simulink model "CHEM_FULL_BENCHMARK"  (R2019a)
settings: Solver=FixedStepAuto  StartTime=0.0  StopTime=app.SimuTime  FixedStep=Te  RelTol=1e-3  EnableMultiTasking=on
values from neighbouring files (symbols this model uses):
  A1 = 0.0154    [INIT_FULL.m]    (also in run.m)
  A2 = 0.0154    [INIT_FULL.m]    (also in run.m)
  app = interface    [INIT_FULL.m]    (also in run.m)
  Cvb = 1.5938*1e-4    (= 0.00015938)    [INIT_FULL.m]    (also in run.m)
  Cvo = 1.59640*1e-4    (= 0.00015964)    [INIT_FULL.m]    (also in run.m)
  g = 9.81    [INIT_FULL.m]    (also in run.m)
  h1c = 0.5    [INIT_FULL.m]    (also in run.m)
  h1c_0 = 0    [INIT_FULL.m]    (also in run.m)
  h1max = 0.6    [INIT_FULL.m]    (also in run.m)
  h2c_0 = 0    [INIT_FULL.m]    (also in Variables_Update.m = app.InitialwaterlevelinT206EditField.Value; run.m)
  h2c_max = 0.11    [INIT_FULL.m]    (also in run.m)
  h2c_min = 0.09    [INIT_FULL.m]    (also in run.m)
  h2max = 0.6    [INIT_FULL.m]    (also in run.m)
  Ki = 5*1e-6    (= 5e-06)    [INIT_FULL.m]    (also in run.m)
  Kp = 1e-3    (= 0.001)    [INIT_FULL.m]    (also in run.m)
  Patm = 101325    [INIT_FULL.m]    (also in run.m)
  Qf1 = 1e-4    (= 0.0001)    [INIT_FULL.m]    (also in Variables_Update.m = app.FlowleakfromT1m3sEditField.Value; run.m)
  Qf2 = 1e-4    (= 0.0001)    [INIT_FULL.m]    (also in Variables_Update.m = app.FlowleakfromT2m3sEditField.Value; run.m)
  Qof1 = 1e-4    (= 0.0001)    [INIT_FULL.m]    (also in Variables_Update.m = app.OverflowrateinT1m3sEditField.Value; run.m)
  Qpmax = 1e-2    (= 0.01)    [INIT_FULL.m]    (also in run.m)
  rate_noise_mQp = 0.01*1e-5    (= 1e-07)    [INIT_FULL.m]    (also in run.m)
  rate_noise_mUp = 0.01*1e-5    (= 1e-07)    [INIT_FULL.m]    (also in run.m)
  rate_noise_my1 = 0.5*0.001    (= 0.0005)    [INIT_FULL.m]    (also in run.m)
  rate_noise_my2 = 0.3*0.001    (= 0.0003)    [INIT_FULL.m]    (also in run.m)
  ro = 1000    [INIT_FULL.m]    (also in run.m)
  seed = randi(10000000)    [INIT_FULL.m]    (also in run.m)
  Te = 1    [INIT_FULL.m]    (also in run.m)
  yo = 0    [INIT_FULL.m]    (also in run.m)
(part 2 of 12)

== system CHEM_FULL_BENCHMARK/T2 hidden long theft/Process ==
  note: y2
  note: y1
  note: Ub
  note: Up
  note: Qvo
      | To users
  note: Qp
  note: Qvb
  Constant : Constant  Value=yo
  Subsystem1 : Subsystem
      mask Display: disp('TANK 1')
  Subsystem10 : Subsystem
      mask Display: disp('Sensor\n y2')
  Subsystem11 : Subsystem
      mask Display: disp('Controller 1')
  Subsystem12 : Subsystem
      mask Display: disp('Sensor\n Ub')
  Subsystem13 : Subsystem
      mask Display: disp('Sensor\n Up')
  Subsystem14 : Subsystem
      mask Display: disp('Sensor\n Qp')
  Subsystem15 : Subsystem
      mask Display: disp('Sensor\n P2')
  Subsystem2 : Subsystem
      mask Display: disp('Valve B')
  Subsystem3 : Subsystem
      mask Display: disp('Valve O')
  Subsystem4 : Subsystem
      mask Display: disp('Controller2')
  Subsystem5 : Subsystem
      mask Display: disp('Sensor\n P1')
  Subsystem6 : Subsystem
      mask Display: disp('Pump')
  Subsystem7 : Subsystem
      mask Display: disp('Sensor\n y1')
  Subsystem8 : Subsystem
      mask Display: disp('TANK 2')
  Subsystem9 : Subsystem
      mask Display: disp('OPERATOR\nSET')
  mQp : Outport
  mUb : Outport  Port=2
  "Uo " : Outport  Port=3
  my1 : Outport  Port=4
  my2 : Outport  Port=5
  h1c : Outport  Port=6
  mUp : Outport  Port=7
  mq0 : Outport  Port=8
  y1 : Outport  Port=9
  vol1 : Outport  Port=10
  y2 : Outport  Port=11
  vol2 : Outport  Port=12
  mP1 : Outport  Port=13
  mP2 : Outport  Port=14
  wires:
  Subsystem12/1(mUb) -> mUb/1
  Subsystem3/1(Qv0) -> mq0/1, Subsystem8/1(Qvo)
  Constant/1 -> Subsystem3/3(y0)
  Subsystem13/1(mUp) -> mUp/1
  Subsystem2/1(QVb) -> Subsystem8/2(Qvb), Subsystem1/2(Qvb)
  Subsystem11/1(mUp) -> Subsystem13/1(Up), Subsystem6/1(Up)
  Subsystem9/1(Out3) -> Subsystem11/1(h1c), h1c/1
  Subsystem9/2(Out1) -> "Uo "/1, Subsystem3/1(U0)
  Subsystem7/1(Out5) -> Subsystem11/2(my1), my1/1
  Subsystem14/1(mQp) -> mQp/1
  Subsystem4/1(Out5) -> Subsystem12/1(Ub), Subsystem2/1(Ub)
  Subsystem10/1(my2) -> my2/1, Subsystem4/1(In2)
  Subsystem6/1(mUp) -> Subsystem1/1(Qp), Subsystem14/1(Qp)
  Subsystem7/2(Out1) -> y1/1
  Subsystem7/3(Out2) -> vol1/1
  Subsystem10/2(yy2) -> y2/1
  Subsystem10/3(vol2) -> vol2/1
  Subsystem5/1(mP1) -> mP1/1
  Subsystem1/1(y1) -> Subsystem5/1(y1), Subsystem2/2(y1), Subsystem7/1(In1)
  Subsystem15/1(mP2) -> mP2/1
  Subsystem8/1(y2) -> Subsystem3/2(y2), Subsystem15/1(y2), Subsystem2/3(y2), Subsystem10/1(y2)

== system CHEM_FULL_BENCHMARK/T2 hidden short theft/Process ==
  note: y2
  note: y1
  note: Ub
  note: Up
  note: Qvo
      | To users
  note: Qp
  note: Qvb
  Constant : Constant  Value=yo
  Subsystem1 : Subsystem
      mask Display: disp('TANK 1')
  Subsystem10 : Subsystem
      mask Display: disp('Sensor\n y2')
  Subsystem11 : Subsystem
      mask Display: disp('Controller 1')
  Subsystem12 : Subsystem
      mask Display: disp('Sensor\n Ub')
  Subsystem13 : Subsystem
      mask Display: disp('Sensor\n Up')
  Subsystem14 : Subsystem
      mask Display: disp('Sensor\n Qp')
  Subsystem15 : Subsystem
      mask Display: disp('Sensor\n P2')
  Subsystem2 : Subsystem
      mask Display: disp('Valve B')
  Subsystem3 : Subsystem
      mask Display: disp('Valve O')
  Subsystem4 : Subsystem
      mask Display: disp('Controller2')
  Subsystem5 : Subsystem
      mask Display: disp('Sensor\n P1')
  Subsystem6 : Subsystem
      mask Display: disp('Pump')
  Subsystem7 : Subsystem
      mask Display: disp('Sensor\n y1')
  Subsystem8 : Subsystem
      mask Display: disp('TANK 2')
  Subsystem9 : Subsystem
      mask Display: disp('OPERATOR\nSET')
  mQp : Outport
  mUb : Outport  Port=2
  "Uo " : Outport  Port=3
  my1 : Outport  Port=4
  my2 : Outport  Port=5
  h1c : Outport  Port=6
  mUp : Outport  Port=7
  mq0 : Outport  Port=8
  y1 : Outport  Port=9
  vol1 : Outport  Port=10
  y2 : Outport  Port=11
  vol2 : Outport  Port=12
  mP1 : Outport  Port=13
  mP2 : Outport  Port=14
  wires:
  Subsystem12/1(mUb) -> mUb/1
  Subsystem3/1(Qv0) -> mq0/1, Subsystem8/1(Qvo)
  Constant/1 -> Subsystem3/3(y0)
  Subsystem13/1(mUp) -> mUp/1
  Subsystem2/1(QVb) -> Subsystem8/2(Qvb), Subsystem1/2(Qvb)
  Subsystem11/1(mUp) -> Subsystem13/1(Up), Subsystem6/1(Up)
  Subsystem9/1(Out3) -> Subsystem11/1(h1c), h1c/1
  Subsystem9/2(Out1) -> "Uo "/1, Subsystem3/1(U0)
  Subsystem7/1(Out5) -> Subsystem11/2(my1), my1/1
  Subsystem14/1(mQp) -> mQp/1
  Subsystem4/1(Out5) -> Subsystem12/1(Ub), Subsystem2/1(Ub)
  Subsystem10/1(my2) -> my2/1, Subsystem4/1(In2)
  Subsystem6/1(mUp) -> Subsystem1/1(Qp), Subsystem14/1(Qp)
  Subsystem7/2(Out1) -> y1/1
  Subsystem7/3(Out2) -> vol1/1
  Subsystem10/2(yy2) -> y2/1
  Subsystem10/3(vol2) -> vol2/1
  Subsystem5/1(mP1) -> mP1/1
  Subsystem1/1(y1) -> Subsystem5/1(y1), Subsystem2/2(y1), Subsystem7/1(In1)
  Subsystem15/1(mP2) -> mP2/1
  Subsystem8/1(y2) -> Subsystem3/2(y2), Subsystem15/1(y2), Subsystem2/3(y2), Subsystem10/1(y2)

== system CHEM_FULL_BENCHMARK/T2 semi hidden long theft/Process ==
  note: y2
  note: y1
  note: Ub
  note: Up
  note: Qvo
      | To users
  note: Qp
  note: Qvb
  Constant : Constant  Value=yo
  Subsystem1 : Subsystem
      mask Display: disp('TANK 1')
  Subsystem10 : Subsystem
      mask Display: disp('Sensor\n y2')
  Subsystem11 : Subsystem
      mask Display: disp('Controller 1')
  Subsystem12 : Subsystem
      mask Display: disp('Sensor\n Ub')
  Subsystem13 : Subsystem
      mask Display: disp('Sensor\n Up')
  Subsystem14 : Subsystem
      mask Display: disp('Sensor\n Qp')
  Subsystem15 : Subsystem
      mask Display: disp('Sensor\n P2')
  Subsystem2 : Subsystem
      mask Display: disp('Valve B')
  Subsystem3 : Subsystem
      mask Display: disp('Valve O')
  Subsystem4 : Subsystem
      mask Display: disp('Controller2')
  Subsystem5 : Subsystem
      mask Display: disp('Sensor\n P1')
  Subsystem6 : Subsystem
      mask Display: disp('Pump')
  Subsystem7 : Subsystem
      mask Display: disp('Sensor\n y1')
  Subsystem8 : Subsystem
      mask Display: disp('TANK 2')
  Subsystem9 : Subsystem
      mask Display: disp('OPERATOR\nSET')
  mQp : Outport
  mUb : Outport  Port=2
  "Uo " : Outport  Port=3
  my1 : Outport  Port=4
  my2 : Outport  Port=5
  h1c : Outport  Port=6
  mUp : Outport  Port=7
  mq0 : Outport  Port=8
  y1 : Outport  Port=9
  vol1 : Outport  Port=10
  y2 : Outport  Port=11
  vol2 : Outport  Port=12
  mP1 : Outport  Port=13
  mP2 : Outport  Port=14
  wires:
  Subsystem12/1(mUb) -> mUb/1
  Subsystem3/1(Qv0) -> mq0/1, Subsystem8/1(Qvo)
  Constant/1 -> Subsystem3/3(y0)
  Subsystem13/1(mUp) -> mUp/1
  Subsystem2/1(QVb) -> Subsystem8/2(Qvb), Subsystem1/2(Qvb)
  Subsystem11/1(mUp) -> Subsystem13/1(Up), Subsystem6/1(Up)
  Subsystem9/1(Out3) -> Subsystem11/1(h1c), h1c/1
  Subsystem9/2(Out1) -> "Uo "/1, Subsystem3/1(U0)
  Subsystem7/1(Out5) -> Subsystem11/2(my1), my1/1
  Subsystem14/1(mQp) -> mQp/1
  Subsystem4/1(Out5) -> Subsystem12/1(Ub), Subsystem2/1(Ub)
  Subsystem10/1(my2) -> my2/1, Subsystem4/1(In2)
  Subsystem6/1(mUp) -> Subsystem1/1(Qp), Subsystem14/1(Qp)
  Subsystem7/2(Out1) -> y1/1
  Subsystem7/3(Out2) -> vol1/1
  Subsystem10/2(yy2) -> y2/1
  Subsystem10/3(vol2) -> vol2/1
  Subsystem5/1(mP1) -> mP1/1
  Subsystem1/1(y1) -> Subsystem5/1(y1), Subsystem2/2(y1), Subsystem7/1(In1)
  Subsystem15/1(mP2) -> mP2/1
  Subsystem8/1(y2) -> Subsystem3/2(y2), Subsystem15/1(y2), Subsystem2/3(y2), Subsystem10/1(y2)

== system CHEM_FULL_BENCHMARK/T2 short theft/Process ==
  note: y2
  note: y1
  note: Ub
  note: Up
  note: Qvo
      | To users
  note: Qp
  note: Qvb
  Constant : Constant  Value=yo
  Subsystem1 : Subsystem
      mask Display: disp('TANK 1')
  Subsystem10 : Subsystem
      mask Display: disp('Sensor\n y2')
  Subsystem11 : Subsystem
      mask Display: disp('Controller 1')
  Subsystem12 : Subsystem
      mask Display: disp('Sensor\n Ub')
  Subsystem13 : Subsystem
      mask Display: disp('Sensor\n Up')
  Subsystem14 : Subsystem
      mask Display: disp('Sensor\n Qp')
  Subsystem15 : Subsystem
      mask Display: disp('Sensor\n P2')
  Subsystem2 : Subsystem
      mask Display: disp('Valve B')
  Subsystem3 : Subsystem
      mask Display: disp('Valve O')
  Subsystem4 : Subsystem
      mask Display: disp('Controller2')
  Subsystem5 : Subsystem
      mask Display: disp('Sensor\n P1')
  Subsystem6 : Subsystem
      mask Display: disp('Pump')
  Subsystem7 : Subsystem
      mask Display: disp('Sensor\n y1')
  Subsystem8 : Subsystem
      mask Display: disp('TANK 2')
  Subsystem9 : Subsystem
      mask Display: disp('OPERATOR\nSET')
  mQp : Outport
  mUb : Outport  Port=2
  "Uo " : Outport  Port=3
  my1 : Outport  Port=4
  my2 : Outport  Port=5
  h1c : Outport  Port=6
  mUp : Outport  Port=7
  mq0 : Outport  Port=8
  y1 : Outport  Port=9
  vol1 : Outport  Port=10
  y2 : Outport  Port=11
  vol2 : Outport  Port=12
  mP1 : Outport  Port=13
  mP2 : Outport  Port=14
  wires:
  Subsystem12/1(mUb) -> mUb/1
  Subsystem3/1(Qv0) -> mq0/1, Subsystem8/1(Qvo)
  Constant/1 -> Subsystem3/3(y0)
  Subsystem13/1(mUp) -> mUp/1
  Subsystem2/1(QVb) -> Subsystem8/2(Qvb), Subsystem1/2(Qvb)
  Subsystem11/1(mUp) -> Subsystem13/1(Up), Subsystem6/1(Up)
  Subsystem9/1(Out3) -> Subsystem11/1(h1c), h1c/1
  Subsystem9/2(Out1) -> "Uo "/1, Subsystem3/1(U0)
  Subsystem7/1(Out5) -> Subsystem11/2(my1), my1/1
  Subsystem14/1(mQp) -> mQp/1
  Subsystem4/1(Out5) -> Subsystem12/1(Ub), Subsystem2/1(Ub)
  Subsystem10/1(my2) -> my2/1, Subsystem4/1(In2)
  Subsystem6/1(mUp) -> Subsystem1/1(Qp), Subsystem14/1(Qp)
  Subsystem7/2(Out1) -> y1/1
  Subsystem7/3(Out2) -> vol1/1
  Subsystem10/2(yy2) -> y2/1
  Subsystem10/3(vol2) -> vol2/1
  Subsystem5/1(mP1) -> mP1/1
  Subsystem1/1(y1) -> Subsystem2/2(y1), Subsystem5/1(y1), Subsystem7/1(In1)
  Subsystem15/1(mP2) -> mP2/1
  Subsystem8/1(y2) -> Subsystem3/2(y2), Subsystem15/1(y2), Subsystem2/3(y2), Subsystem10/1(y2)

== system CHEM_FULL_BENCHMARK/Theft when no use/Process ==
  note: y2
  note: y1
  note: Ub
  note: Up
  note: Qvo
      | To users
  note: Qp
  note: Qvb
  Constant : Constant  Value=yo
  Subsystem1 : Subsystem
      mask Display: disp('TANK 1')
  Subsystem10 : Subsystem
      mask Display: disp('Sensor\n y2')
  Subsystem11 : Subsystem
      mask Display: disp('Controller 1')
  Subsystem12 : Subsystem
      mask Display: disp('Sensor\n Ub')
  Subsystem13 : Subsystem
      mask Display: disp('Sensor\n Up')
  Subsystem14 : Subsystem
      mask Display: disp('Sensor\n Qp')
  Subsystem15 : Subsystem
      mask Display: disp('Sensor\n P2')
  Subsystem2 : Subsystem
      mask Display: disp('Valve B')
  Subsystem3 : Subsystem
      mask Display: disp('Valve O')
  Subsystem4 : Subsystem
      mask Display: disp('Controller2')
  Subsystem5 : Subsystem
      mask Display: disp('Sensor\n P1')
  Subsystem6 : Subsystem
      mask Display: disp('Pump')
  Subsystem7 : Subsystem
      mask Display: disp('Sensor\n y1')
  Subsystem8 : Subsystem
      mask Display: disp('TANK 2')
  Subsystem9 : Subsystem
      mask Display: disp('OPERATOR\nSET')
  mQp : Outport
  mUb : Outport  Port=2
  "Uo " : Outport  Port=3
  my1 : Outport  Port=4
  my2 : Outport  Port=5
  h1c : Outport  Port=6
  mUp : Outport  Port=7
  mq0 : Outport  Port=8
  y1 : Outport  Port=9
  vol1 : Outport  Port=10
  y2 : Outport  Port=11
  vol2 : Outport  Port=12
  mP1 : Outport  Port=13
  mP2 : Outport  Port=14
  wires:
  Subsystem12/1(mUb) -> mUb/1
  Subsystem3/1(Qv0) -> mq0/1, Subsystem8/1(Qvo)
  Constant/1 -> Subsystem3/3(y0)
  Subsystem13/1(mUp) -> mUp/1
  Subsystem8/1(y2) -> Subsystem10/1(y2), Subsystem15/1(y2), Subsystem2/3(y2), Subsystem3/2(y2)
  Subsystem2/1(QVb) -> Subsystem8/2(Qvb), Subsystem1/2(Qvb)
  Subsystem11/1(mUp) -> Subsystem13/1(Up), Subsystem6/1(Up)
  Subsystem9/1(Out3) -> Subsystem11/1(h1c), h1c/1
  Subsystem7/1(Out5) -> Subsystem11/2(my1), my1/1
  Subsystem14/1(mQp) -> mQp/1
  Subsystem4/1(Out5) -> Subsystem12/1(Ub), Subsystem2/1(Ub)
  Subsystem10/1(my2) -> my2/1, Subsystem4/1(In2)
  Subsystem6/1(mUp) -> Subsystem1/1(Qp), Subsystem14/1(Qp)
  Subsystem7/2(Out1) -> y1/1
  Subsystem7/3(Out2) -> vol1/1
  Subsystem10/2(yy2) -> y2/1
  Subsystem10/3(vol2) -> vol2/1
  Subsystem5/1(mP1) -> mP1/1
  Subsystem1/1(y1) -> Subsystem5/1(y1), Subsystem2/2(y1), Subsystem7/1(In1)
  Subsystem15/1(mP2) -> mP2/1
  Subsystem9/2(Out1) -> "Uo "/1, Subsystem8/3(U0), Subsystem3/1(U0)

== system CHEM_FULL_BENCHMARK/Theft when no use same rate as user/Process ==
  note: y2
  note: y1
  note: Ub
  note: Up
  note: Qvo
      | To users
  note: Qp
  note: Qvb
  Constant : Constant  Value=yo
  Subsystem1 : Subsystem
      mask Display: disp('TANK 1')
  Subsystem10 : Subsystem
      mask Display: disp('Sensor\n y2')
  Subsystem11 : Subsystem
      mask Display: disp('Controller 1')
  Subsystem12 : Subsystem
      mask Display: disp('Sensor\n Ub')
  Subsystem13 : Subsystem
      mask Display: disp('Sensor\n Up')
  Subsystem14 : Subsystem
      mask Display: disp('Sensor\n Qp')
  Subsystem15 : Subsystem
      mask Display: disp('Sensor\n P2')
  Subsystem2 : Subsystem
      mask Display: disp('Valve B')
  Subsystem3 : Subsystem
      mask Display: disp('Valve O')
  Subsystem4 : Subsystem
      mask Display: disp('Controller2')
  Subsystem5 : Subsystem
      mask Display: disp('Sensor\n P1')
  Subsystem6 : Subsystem
      mask Display: disp('Pump')
  Subsystem7 : Subsystem
      mask Display: disp('Sensor\n y1')
  Subsystem8 : Subsystem
      mask Display: disp('TANK 2')
  Subsystem9 : Subsystem
      mask Display: disp('OPERATOR\nSET')
  mQp : Outport
  mUb : Outport  Port=2
  "Uo " : Outport  Port=3
  my1 : Outport  Port=4
  my2 : Outport  Port=5
  h1c : Outport  Port=6
  mUp : Outport  Port=7
  mq0 : Outport  Port=8
  y1 : Outport  Port=9
  vol1 : Outport  Port=10
  y2 : Outport  Port=11
  vol2 : Outport  Port=12
  mP1 : Outport  Port=13
  mP2 : Outport  Port=14
  wires:
  Subsystem12/1(mUb) -> mUb/1
  Subsystem3/1(Qv0) -> mq0/1, Subsystem8/1(Qvo)
  Constant/1 -> Subsystem3/3(y0)
  Subsystem13/1(mUp) -> mUp/1
  Subsystem2/1(QVb) -> Subsystem8/2(Qvb), Subsystem1/2(Qvb)
  Subsystem11/1(mUp) -> Subsystem13/1(Up), Subsystem6/1(Up)
  Subsystem9/1(Out3) -> Subsystem11/1(h1c), h1c/1
  Subsystem9/2(Out1) -> "Uo "/1, Subsystem8/3(U0), Subsystem3/1(U0)
  Subsystem7/1(Out5) -> Subsystem11/2(my1), my1/1
  Subsystem14/1(mQp) -> mQp/1
  Subsystem4/1(Out5) -> Subsystem2/1(Ub), Subsystem12/1(Ub)
  Subsystem10/1(my2) -> my2/1, Subsystem8/4(my2), Subsystem4/1(In2)
  Subsystem6/1(mUp) -> Subsystem1/1(Qp), Subsystem14/1(Qp)
  Subsystem7/2(Out1) -> y1/1
  Subsystem7/3(Out2) -> vol1/1
  Subsystem10/2(yy2) -> y2/1
  Subsystem10/3(vol2) -> vol2/1
  Subsystem5/1(mP1) -> mP1/1
  Subsystem1/1(y1) -> Subsystem5/1(y1), Subsystem2/2(y1), Subsystem7/1(In1)
  Subsystem15/1(mP2) -> mP2/1
  Subsystem8/1(y2) -> Subsystem10/1(y2), Subsystem15/1(y2), Subsystem2/3(y2), Subsystem3/2(y2)

== system CHEM_FULL_BENCHMARK/Vb fault/Process ==
  note: y2
  note: y1
  note: Ub
  note: Up
  note: Qvo
      | To users
  note: Qp
  note: Qvb
  Constant : Constant  Value=yo
  Subsystem1 : Subsystem
      mask Display: disp('TANK 1')
  Subsystem10 : Subsystem
      mask Display: disp('Sensor\n y2')
  Subsystem11 : Subsystem
      mask Display: disp('Controller 1')
  Subsystem12 : Subsystem
      mask Display: disp('Sensor\n Ub')
  Subsystem13 : Subsystem
      mask Display: disp('Sensor\n Up')
  Subsystem14 : Subsystem
      mask Display: disp('Sensor\n Qp')
  Subsystem15 : Subsystem
      mask Display: disp('Sensor\n P2')
  Subsystem2 : Subsystem
      mask Display: disp('Valve B')
  Subsystem3 : Subsystem
      mask Display: disp('Valve O')
  Subsystem4 : Subsystem
      mask Display: disp('Controller2')
  Subsystem5 : Subsystem
      mask Display: disp('Sensor\n P1')
  Subsystem6 : Subsystem
      mask Display: disp('Pump')
  Subsystem7 : Subsystem
      mask Display: disp('Sensor\n y1')
  Subsystem8 : Subsystem
      mask Display: disp('TANK 2')
  Subsystem9 : Subsystem
      mask Display: disp('OPERATOR\nSET')
  mQp : Outport
  mUb : Outport  Port=2
  "Uo " : Outport  Port=3
  my1 : Outport  Port=4
  my2 : Outport  Port=5
  h1c : Outport  Port=6
  mUp : Outport  Port=7
  mq0 : Outport  Port=8
  y1 : Outport  Port=9
  vol1 : Outport  Port=10
  y2 : Outport  Port=11
  vol2 : Outport  Port=12
  mP1 : Outport  Port=13
  mP2 : Outport  Port=14
  wires:
  Subsystem12/1(mUb) -> mUb/1
  Subsystem3/1(Qv0) -> mq0/1, Subsystem8/1(Qvo)
  Constant/1 -> Subsystem3/3(y0)
  Subsystem13/1(mUp) -> mUp/1
  Subsystem2/1(QVb) -> Subsystem8/2(Qvb), Subsystem1/2(Qvb)
  Subsystem11/1(mUp) -> Subsystem13/1(Up), Subsystem6/1(Up)
  Subsystem9/1(Out3) -> Subsystem11/1(h1c), h1c/1
  Subsystem9/2(Out1) -> "Uo "/1, Subsystem3/1(U0)
  Subsystem7/1(Out5) -> Subsystem11/2(my1), my1/1
  Subsystem14/1(mQp) -> mQp/1
  Subsystem4/1(Out5) -> Subsystem12/1(Ub), Subsystem2/1(Ub)
  Subsystem10/1(my2) -> my2/1, Subsystem4/1(In2)
  Subsystem6/1(mUp) -> Subsystem1/1(Qp), Subsystem14/1(Qp)
  Subsystem7/2(Out1) -> y1/1
  Subsystem7/3(Out2) -> vol1/1
  Subsystem10/2(yy2) -> y2/1
  Subsystem10/3(vol2) -> vol2/1
  Subsystem5/1(mP1) -> mP1/1
  Subsystem1/1(y1) -> Subsystem5/1(y1), Subsystem2/2(y1), Subsystem7/1(In1)
  Subsystem15/1(mP2) -> mP2/1
  Subsystem8/1(y2) -> Subsystem3/2(y2), Subsystem15/1(y2), Subsystem2/3(y2), Subsystem10/1(y2)

== system CHEM_FULL_BENCHMARK/faultless/Process ==
  note: y2
  note: y1
  note: Ub
  note: Up
  note: Qvo
      | To users
  note: Qp
  note: Qvb
  Constant : Constant  Value=yo
  Subsystem1 : Subsystem
      mask Display: disp('TANK 1')
  Subsystem10 : Subsystem
      mask Display: disp('Sensor\n y2')
  Subsystem11 : Subsystem
      mask Display: disp('Controller 1')
  Subsystem12 : Subsystem
      mask Display: disp('Sensor\n Ub')
  Subsystem13 : Subsystem
      mask Display: disp('Sensor\n Up')
  Subsystem14 : Subsystem
      mask Display: disp('Sensor\n Qp')
  Subsystem15 : Subsystem
      mask Display: disp('Sensor\n P2')
  Subsystem2 : Subsystem
      mask Display: disp('Valve B')
  Subsystem3 : Subsystem
      mask Display: disp('Valve O')
  Subsystem4 : Subsystem
      mask Display: disp('Controller2')
  Subsystem5 : Subsystem
      mask Display: disp('Sensor\n P1')
  Subsystem6 : Subsystem
      mask Display: disp('Pump')
  Subsystem7 : Subsystem
      mask Display: disp('Sensor\n y1')
  Subsystem8 : Subsystem
      mask Display: disp('TANK 2')
  Subsystem9 : Subsystem
      mask Display: disp('OPERATOR\nSET')
  mQp : Outport
  mUb : Outport  Port=2
  "Uo " : Outport  Port=3
  my1 : Outport  Port=4
  my2 : Outport  Port=5
  h1c : Outport  Port=6
  mUp : Outport  Port=7
  mq0 : Outport  Port=8
  y1 : Outport  Port=9
  vol1 : Outport  Port=10
  y2 : Outport  Port=11
  vol2 : Outport  Port=12
  mP1 : Outport  Port=13
  mP2 : Outport  Port=14
  wires:
  Subsystem1/1(y1) -> Subsystem5/1(y1), Subsystem2/2(y1), Subsystem7/1(In1)
  Subsystem12/1(mUb) -> mUb/1
  Subsystem3/1(Qv0) -> mq0/1, Subsystem8/1(Qvo)
  Constant/1 -> Subsystem3/3(y0)
  Subsystem13/1(mUp) -> mUp/1
  Subsystem8/1(y2) -> Subsystem3/2(y2), Subsystem15/1(y2), Subsystem2/3(y2), Subsystem10/1(y2)
  Subsystem2/1(QVb) -> Subsystem8/2(Qvb), Subsystem1/2(Qvb)
  Subsystem11/1(mUp) -> Subsystem13/1(Up), Subsystem6/1(Up)
  Subsystem9/1(Out3) -> Subsystem11/1(h1c), h1c/1
  Subsystem9/2(Out1) -> "Uo "/1, Subsystem3/1(U0)
  Subsystem7/1(Out5) -> Subsystem11/2(my1), my1/1
  Subsystem14/1(mQp) -> mQp/1
  Subsystem4/1(Out5) -> Subsystem12/1(Ub), Subsystem2/1(Ub)
  Subsystem10/1(my2) -> my2/1, Subsystem4/1(In2)
  Subsystem6/1(mUp) -> Subsystem1/1(Qp), Subsystem14/1(Qp)
  Subsystem7/2(Out1) -> y1/1
  Subsystem7/3(Out2) -> vol1/1
  Subsystem10/2(yy2) -> y2/1
  Subsystem10/3(vol2) -> vol2/1
  Subsystem5/1(mP1) -> mP1/1
  Subsystem15/1(mP2) -> mP2/1

== system CHEM_FULL_BENCHMARK/faultless1/Process ==
  note: y2
  note: y1
  note: Ub
  note: Up
  note: Qvo
      | To users
  note: Qp
  note: Qvb
  Constant : Constant  Value=yo
  Subsystem1 : Subsystem
      mask Display: disp('TANK 1')
  Subsystem10 : Subsystem
      mask Display: disp('Sensor\n y2')
  Subsystem11 : Subsystem
      mask Display: disp('Controller 1')
  Subsystem12 : Subsystem
      mask Display: disp('Sensor\n Ub')
  Subsystem13 : Subsystem
      mask Display: disp('Sensor\n Up')
  Subsystem14 : Subsystem
      mask Display: disp('Sensor\n Qp')
  Subsystem15 : Subsystem
      mask Display: disp('Sensor\n P2')
  Subsystem2 : Subsystem
      mask Display: disp('Valve B')
  Subsystem3 : Subsystem
      mask Display: disp('Valve O')
  Subsystem4 : Subsystem
      mask Display: disp('Controller2')
  Subsystem5 : Subsystem
      mask Display: disp('Sensor\n P1')
  Subsystem6 : Subsystem
      mask Display: disp('Pump')
  Subsystem7 : Subsystem
      mask Display: disp('Sensor\n y1')
  Subsystem8 : Subsystem
      mask Display: disp('TANK 2')
  Subsystem9 : Subsystem
      mask Display: disp('OPERATOR\nSET')
  mQp : Outport
  mUb : Outport  Port=2
  "Uo " : Outport  Port=3
  my1 : Outport  Port=4
  my2 : Outport  Port=5
  h1c : Outport  Port=6
  mUp : Outport  Port=7
  mq0 : Outport  Port=8
  y1 : Outport  Port=9
  vol1 : Outport  Port=10
  y2 : Outport  Port=11
  vol2 : Outport  Port=12
  mP1 : Outport  Port=13
  mP2 : Outport  Port=14
  wires:
  Subsystem12/1(mUb) -> mUb/1
  Subsystem3/1(Qv0) -> mq0/1, Subsystem8/1(Qvo)
  Constant/1 -> Subsystem3/3(y0)
  Subsystem13/1(mUp) -> mUp/1
  Subsystem2/1(QVb) -> Subsystem8/2(Qvb), Subsystem1/2(Qvb)
  Subsystem11/1(mUp) -> Subsystem13/1(Up), Subsystem6/1(Up)
  Subsystem9/1(Out3) -> Subsystem11/1(h1c), h1c/1
  Subsystem9/2(Out1) -> "Uo "/1, Subsystem3/1(U0)
  Subsystem7/1(Out5) -> Subsystem11/2(my1), my1/1
  Subsystem14/1(mQp) -> mQp/1
  Subsystem4/1(Out5) -> Subsystem12/1(Ub), Subsystem2/1(Ub)
  Subsystem10/1(my2) -> my2/1, Subsystem4/1(In2)
  Subsystem6/1(mUp) -> Subsystem1/1(Qp), Subsystem14/1(Qp)
  Subsystem7/2(Out1) -> y1/1
  Subsystem7/3(Out2) -> vol1/1
  Subsystem10/2(yy2) -> y2/1
  Subsystem10/3(vol2) -> vol2/1
  Subsystem5/1(mP1) -> mP1/1
  Subsystem1/1(y1) -> Subsystem5/1(y1), Subsystem2/2(y1), Subsystem7/1(In1)
  Subsystem15/1(mP2) -> mP2/1
  Subsystem8/1(y2) -> Subsystem3/2(y2), Subsystem15/1(y2), Subsystem2/3(y2), Subsystem10/1(y2)

== system CHEM_FULL_BENCHMARK/faultless2/Process ==
  note: y2
  note: y1
  note: Ub
  note: Up
  note: Qvo
      | To users
  note: Qp
  note: Qvb
  Constant : Constant  Value=yo
  Subsystem1 : Subsystem
      mask Display: disp('TANK 1')
  Subsystem10 : Subsystem
      mask Display: disp('Sensor\n y2')
  Subsystem11 : Subsystem
      mask Display: disp('Controller 1')
  Subsystem12 : Subsystem
      mask Display: disp('Sensor\n Ub')
  Subsystem13 : Subsystem
      mask Display: disp('Sensor\n Up')
  Subsystem14 : Subsystem
      mask Display: disp('Sensor\n Qp')
  Subsystem15 : Subsystem
      mask Display: disp('Sensor\n P2')
  Subsystem2 : Subsystem
      mask Display: disp('Valve B')
  Subsystem3 : Subsystem
      mask Display: disp('Valve O')
  Subsystem4 : Subsystem
      mask Display: disp('Controller2')
  Subsystem5 : Subsystem
      mask Display: disp('Sensor\n P1')
  Subsystem6 : Subsystem
      mask Display: disp('Pump')
  Subsystem7 : Subsystem
      mask Display: disp('Sensor\n y1')
  Subsystem8 : Subsystem
      mask Display: disp('TANK 2')
  Subsystem9 : Subsystem
      mask Display: disp('OPERATOR\nSET')
  mQp : Outport
  mUb : Outport  Port=2
  "Uo " : Outport  Port=3
  my1 : Outport  Port=4
  my2 : Outport  Port=5
  h1c : Outport  Port=6
  mUp : Outport  Port=7
  mq0 : Outport  Port=8
  y1 : Outport  Port=9
  vol1 : Outport  Port=10
  y2 : Outport  Port=11
  vol2 : Outport  Port=12
  mP1 : Outport  Port=13
  mP2 : Outport  Port=14
  wires:
  Subsystem12/1(mUb) -> mUb/1
  Subsystem3/1(Qv0) -> mq0/1, Subsystem8/1(Qvo)
  Constant/1 -> Subsystem3/3(y0)
  Subsystem13/1(mUp) -> mUp/1
  Subsystem2/1(QVb) -> Subsystem8/2(Qvb), Subsystem1/2(Qvb)
  Subsystem11/1(mUp) -> Subsystem13/1(Up), Subsystem6/1(Up)
  Subsystem9/1(Out3) -> Subsystem11/1(h1c), h1c/1
  Subsystem9/2(Out1) -> "Uo "/1, Subsystem3/1(U0)
  Subsystem7/1(Out5) -> Subsystem11/2(my1), my1/1
  Subsystem14/1(mQp) -> mQp/1
  Subsystem4/1(Out5) -> Subsystem12/1(Ub), Subsystem2/1(Ub)
  Subsystem10/1(my2) -> my2/1, Subsystem4/1(In2)
  Subsystem6/1(mUp) -> Subsystem1/1(Qp), Subsystem14/1(Qp)
  Subsystem7/2(Out1) -> y1/1
  Subsystem7/3(Out2) -> vol1/1
  Subsystem10/2(yy2) -> y2/1
  Subsystem10/3(vol2) -> vol2/1
  Subsystem5/1(mP1) -> mP1/1
  Subsystem1/1(y1) -> Subsystem5/1(y1), Subsystem2/2(y1), Subsystem7/1(In1)
  Subsystem15/1(mP2) -> mP2/1
  Subsystem8/1(y2) -> Subsystem3/2(y2), Subsystem15/1(y2), Subsystem2/3(y2), Subsystem10/1(y2)

== system CHEM_FULL_BENCHMARK/faultless3/Process ==
  note: y2
  note: y1
  note: Ub
  note: Up
  note: Qvo
      | To users
  note: Qp
  note: Qvb
  Constant : Constant  Value=yo
  Subsystem1 : Subsystem
      mask Display: disp('TANK 1')
  Subsystem10 : Subsystem
      mask Display: disp('Sensor\n y2')
  Subsystem11 : Subsystem
      mask Display: disp('Controller 1')
  Subsystem12 : Subsystem
      mask Display: disp('Sensor\n Ub')
  Subsystem13 : Subsystem
      mask Display: disp('Sensor\n Up')
  Subsystem14 : Subsystem
      mask Display: disp('Sensor\n Qp')
  Subsystem15 : Subsystem
      mask Display: disp('Sensor\n P2')
  Subsystem2 : Subsystem
      mask Display: disp('Valve B')
  Subsystem3 : Subsystem
      mask Display: disp('Valve O')
  Subsystem4 : Subsystem
      mask Display: disp('Controller2')
  Subsystem5 : Subsystem
      mask Display: disp('Sensor\n P1')
  Subsystem6 : Subsystem
      mask Display: disp('Pump')
  Subsystem7 : Subsystem
      mask Display: disp('Sensor\n y1')
  Subsystem8 : Subsystem
      mask Display: disp('TANK 2')
  Subsystem9 : Subsystem
      mask Display: disp('OPERATOR\nSET')
  mQp : Outport
  mUb : Outport  Port=2
  "Uo " : Outport  Port=3
  my1 : Outport  Port=4
  my2 : Outport  Port=5
  h1c : Outport  Port=6
  mUp : Outport  Port=7
  mq0 : Outport  Port=8
  y1 : Outport  Port=9
  vol1 : Outport  Port=10
  y2 : Outport  Port=11
  vol2 : Outport  Port=12
  mP1 : Outport  Port=13
  mP2 : Outport  Port=14
  wires:
  Subsystem12/1(mUb) -> mUb/1
  Subsystem3/1(Qv0) -> mq0/1, Subsystem8/1(Qvo)
  Constant/1 -> Subsystem3/3(y0)
  Subsystem13/1(mUp) -> mUp/1
  Subsystem2/1(QVb) -> Subsystem8/2(Qvb), Subsystem1/2(Qvb)
  Subsystem11/1(mUp) -> Subsystem13/1(Up), Subsystem6/1(Up)
  Subsystem9/1(Out3) -> Subsystem11/1(h1c), h1c/1
  Subsystem9/2(Out1) -> "Uo "/1, Subsystem3/1(U0)
  Subsystem7/1(Out5) -> Subsystem11/2(my1), my1/1
  Subsystem14/1(mQp) -> mQp/1
  Subsystem4/1(Out5) -> Subsystem12/1(Ub), Subsystem2/1(Ub)
  Subsystem10/1(my2) -> my2/1, Subsystem4/1(In2)
  Subsystem6/1(mUp) -> Subsystem1/1(Qp), Subsystem14/1(Qp)
  Subsystem7/2(Out1) -> y1/1
  Subsystem7/3(Out2) -> vol1/1
  Subsystem10/2(yy2) -> y2/1
  Subsystem10/3(vol2) -> vol2/1
  Subsystem5/1(mP1) -> mP1/1
  Subsystem1/1(y1) -> Subsystem5/1(y1), Subsystem2/2(y1), Subsystem7/1(In1)
  Subsystem15/1(mP2) -> mP2/1
  Subsystem8/1(y2) -> Subsystem3/2(y2), Subsystem15/1(y2), Subsystem2/3(y2), Subsystem10/1(y2)

== system CHEM_FULL_BENCHMARK/faultless4/Process ==
  note: y2
  note: y1
  note: Ub
  note: Up
  note: Qvo
      | To users
  note: Qp
  note: Qvb
  Constant : Constant  Value=yo
  Subsystem1 : Subsystem
      mask Display: disp('TANK 1')
  Subsystem10 : Subsystem
      mask Display: disp('Sensor\n y2')
  Subsystem11 : Subsystem
      mask Display: disp('Controller 1')
  Subsystem12 : Subsystem
      mask Display: disp('Sensor\n Ub')
  Subsystem13 : Subsystem
      mask Display: disp('Sensor\n Up')
  Subsystem14 : Subsystem
      mask Display: disp('Sensor\n Qp')
  Subsystem15 : Subsystem
      mask Display: disp('Sensor\n P2')
  Subsystem2 : Subsystem
      mask Display: disp('Valve B')
  Subsystem3 : Subsystem
      mask Display: disp('Valve O')
  Subsystem4 : Subsystem
      mask Display: disp('Controller2')
  Subsystem5 : Subsystem
      mask Display: disp('Sensor\n P1')
  Subsystem6 : Subsystem
      mask Display: disp('Pump')
  Subsystem7 : Subsystem
      mask Display: disp('Sensor\n y1')
  Subsystem8 : Subsystem
      mask Display: disp('TANK 2')
  Subsystem9 : Subsystem
      mask Display: disp('OPERATOR\nSET')
  mQp : Outport
  mUb : Outport  Port=2
  "Uo " : Outport  Port=3
  my1 : Outport  Port=4
  my2 : Outport  Port=5
  h1c : Outport  Port=6
  mUp : Outport  Port=7
  mq0 : Outport  Port=8
  y1 : Outport  Port=9
  vol1 : Outport  Port=10
  y2 : Outport  Port=11
  vol2 : Outport  Port=12
  mP1 : Outport  Port=13
  mP2 : Outport  Port=14
  wires:
  Subsystem12/1(mUb) -> mUb/1
  Subsystem3/1(Qv0) -> mq0/1, Subsystem8/1(Qvo)
  Constant/1 -> Subsystem3/3(y0)
  Subsystem13/1(mUp) -> mUp/1
  Subsystem2/1(QVb) -> Subsystem8/2(Qvb), Subsystem1/2(Qvb)
  Subsystem11/1(mUp) -> Subsystem13/1(Up), Subsystem6/1(Up)
  Subsystem9/1(Out3) -> Subsystem11/1(h1c), h1c/1
  Subsystem9/2(Out1) -> "Uo "/1, Subsystem3/1(U0)
  Subsystem7/1(Out5) -> Subsystem11/2(my1), my1/1
  Subsystem14/1(mQp) -> mQp/1
  Subsystem4/1(Out5) -> Subsystem12/1(Ub), Subsystem2/1(Ub)
  Subsystem10/1(my2) -> my2/1, Subsystem4/1(In2)
  Subsystem6/1(mUp) -> Subsystem1/1(Qp), Subsystem14/1(Qp)
  Subsystem7/2(Out1) -> y1/1
  Subsystem7/3(Out2) -> vol1/1
  Subsystem10/2(yy2) -> y2/1
  Subsystem10/3(vol2) -> vol2/1
  Subsystem5/1(mP1) -> mP1/1
  Subsystem1/1(y1) -> Subsystem5/1(y1), Subsystem2/2(y1), Subsystem7/1(In1)
  Subsystem15/1(mP2) -> mP2/1
  Subsystem8/1(y2) -> Subsystem3/2(y2), Subsystem15/1(y2), Subsystem2/3(y2), Subsystem10/1(y2)

== system CHEM_FULL_BENCHMARK/mUb fault/Process ==
  note: y2
  note: y1
  note: Ub
  note: Up
  note: Qvo
      | To users
  note: Qp
  note: Qvb
  Constant : Constant  Value=yo
  Subsystem1 : Subsystem
      mask Display: disp('TANK 1')
  Subsystem10 : Subsystem
      mask Display: disp('Sensor\n y2')
  Subsystem11 : Subsystem
      mask Display: disp('Controller 1')
  Subsystem12 : Subsystem
      mask Display: disp('Sensor\n Ub')
  Subsystem13 : Subsystem
      mask Display: disp('Sensor\n Up')
  Subsystem14 : Subsystem
      mask Display: disp('Sensor\n Qp')
  Subsystem15 : Subsystem
      mask Display: disp('Sensor\n P2')
  Subsystem2 : Subsystem
      mask Display: disp('Valve B')
  Subsystem3 : Subsystem
      mask Display: disp('Valve O')
  Subsystem4 : Subsystem
      mask Display: disp('Controller2')
  Subsystem5 : Subsystem
      mask Display: disp('Sensor\n P1')
  Subsystem6 : Subsystem
      mask Display: disp('Pump')
  Subsystem7 : Subsystem
      mask Display: disp('Sensor\n y1')
  Subsystem8 : Subsystem
      mask Display: disp('TANK 2')
  Subsystem9 : Subsystem
      mask Display: disp('OPERATOR\nSET')
  mQp : Outport
  mUb : Outport  Port=2
  "Uo " : Outport  Port=3
  my1 : Outport  Port=4
  my2 : Outport  Port=5
  h1c : Outport  Port=6
  mUp : Outport  Port=7
  mq0 : Outport  Port=8
  y1 : Outport  Port=9
  vol1 : Outport  Port=10
  y2 : Outport  Port=11
  vol2 : Outport  Port=12
  mP1 : Outport  Port=13
  mP2 : Outport  Port=14
  wires:
  Subsystem12/1(mUb) -> mUb/1
  Subsystem3/1(Qv0) -> mq0/1, Subsystem8/1(Qvo)
  Constant/1 -> Subsystem3/3(y0)
  Subsystem13/1(mUp) -> mUp/1
  Subsystem2/1(QVb) -> Subsystem8/2(Qvb), Subsystem1/2(Qvb)
  Subsystem11/1(mUp) -> Subsystem13/1(Up), Subsystem6/1(Up)
  Subsystem9/1(Out3) -> Subsystem11/1(h1c), h1c/1
  Subsystem9/2(Out1) -> "Uo "/1, Subsystem3/1(U0)
  Subsystem7/1(Out5) -> Subsystem11/2(my1), my1/1
  Subsystem14/1(mQp) -> mQp/1
  Subsystem4/1(Out5) -> Subsystem12/1(Ub), Subsystem2/1(Ub)
  Subsystem10/1(my2) -> my2/1, Subsystem4/1(In2)
  Subsystem6/1(mUp) -> Subsystem1/1(Qp), Subsystem14/1(Qp)
  Subsystem7/2(Out1) -> y1/1
  Subsystem7/3(Out2) -> vol1/1
  Subsystem10/2(yy2) -> y2/1
  Subsystem10/3(vol2) -> vol2/1
  Subsystem5/1(mP1) -> mP1/1
  Subsystem1/1(y1) -> Subsystem5/1(y1), Subsystem2/2(y1), Subsystem7/1(In1)
  Subsystem15/1(mP2) -> mP2/1
  Subsystem8/1(y2) -> Subsystem3/2(y2), Subsystem15/1(y2), Subsystem2/3(y2), Subsystem10/1(y2)

== system CHEM_FULL_BENCHMARK/mUp fault/Process ==
  note: y2
  note: y1
  note: Ub
  note: Up
  note: Qvo
      | To users
  note: Qp
  note: Qvb
  Constant : Constant  Value=yo
  Subsystem1 : Subsystem
      mask Display: disp('TANK 1')
  Subsystem10 : Subsystem
      mask Display: disp('Sensor\n y2')
  Subsystem11 : Subsystem
      mask Display: disp('Controller 1')
  Subsystem12 : Subsystem
      mask Display: disp('Sensor\n Ub')
  Subsystem13 : Subsystem
      mask Display: disp('Sensor\n Up')
  Subsystem14 : Subsystem
      mask Display: disp('Sensor\n Qp')
  Subsystem15 : Subsystem
      mask Display: disp('Sensor\n P2')
  Subsystem2 : Subsystem
      mask Display: disp('Valve B')
  Subsystem3 : Subsystem
      mask Display: disp('Valve O')
  Subsystem4 : Subsystem
      mask Display: disp('Controller2')
  Subsystem5 : Subsystem
      mask Display: disp('Sensor\n P1')
  Subsystem6 : Subsystem
      mask Display: disp('Pump')
  Subsystem7 : Subsystem
      mask Display: disp('Sensor\n y1')
  Subsystem8 : Subsystem
      mask Display: disp('TANK 2')
  Subsystem9 : Subsystem
      mask Display: disp('OPERATOR\nSET')
  mQp : Outport
  mUb : Outport  Port=2
  "Uo " : Outport  Port=3
  my1 : Outport  Port=4
  my2 : Outport  Port=5
  h1c : Outport  Port=6
  mUp : Outport  Port=7
  mq0 : Outport  Port=8
  y1 : Outport  Port=9
  vol1 : Outport  Port=10
  y2 : Outport  Port=11
  vol2 : Outport  Port=12
  mP1 : Outport  Port=13
  mP2 : Outport  Port=14
  wires:
  Subsystem12/1(mUb) -> mUb/1
  Subsystem3/1(Qv0) -> mq0/1, Subsystem8/1(Qvo)
  Constant/1 -> Subsystem3/3(y0)
  Subsystem13/1(mUp) -> mUp/1
  Subsystem2/1(QVb) -> Subsystem8/2(Qvb), Subsystem1/2(Qvb)
  Subsystem11/1(mUp) -> Subsystem13/1(Up), Subsystem6/1(Up)
  Subsystem9/1(Out3) -> Subsystem11/1(h1c), h1c/1
  Subsystem9/2(Out1) -> "Uo "/1, Subsystem3/1(U0)
  Subsystem7/1(Out5) -> Subsystem11/2(my1), my1/1
  Subsystem14/1(mQp) -> mQp/1
  Subsystem4/1(Out5) -> Subsystem12/1(Ub), Subsystem2/1(Ub)
  Subsystem10/1(my2) -> my2/1, Subsystem4/1(In2)
  Subsystem6/1(mUp) -> Subsystem1/1(Qp), Subsystem14/1(Qp)
  Subsystem7/2(Out1) -> y1/1
  Subsystem7/3(Out2) -> vol1/1
  Subsystem10/2(yy2) -> y2/1
  Subsystem10/3(vol2) -> vol2/1
  Subsystem5/1(mP1) -> mP1/1
  Subsystem1/1(y1) -> Subsystem5/1(y1), Subsystem2/2(y1), Subsystem7/1(In1)
  Subsystem15/1(mP2) -> mP2/1
  Subsystem8/1(y2) -> Subsystem3/2(y2), Subsystem2/3(y2), Subsystem15/1(y2), Subsystem10/1(y2)

== system CHEM_FULL_BENCHMARK/my1 fault/Process ==
  note: y2
  note: y1
  note: Ub
  note: Up
  note: Qvo
      | To users
  note: Qp
  note: Qvb
  Constant : Constant  Value=yo
  Subsystem1 : Subsystem
      mask Display: disp('TANK 1')
  Subsystem10 : Subsystem
      mask Display: disp('Sensor\n y2')
  Subsystem11 : Subsystem
      mask Display: disp('Controller 1')
  Subsystem12 : Subsystem
      mask Display: disp('Sensor\n Ub')
  Subsystem13 : Subsystem
      mask Display: disp('Sensor\n Up')
  Subsystem14 : Subsystem
      mask Display: disp('Sensor\n Qp')
  Subsystem15 : Subsystem
      mask Display: disp('Sensor\n P2')
  Subsystem2 : Subsystem
      mask Display: disp('Valve B')
  Subsystem3 : Subsystem
      mask Display: disp('Valve O')
  Subsystem4 : Subsystem
      mask Display: disp('Controller2')
  Subsystem5 : Subsystem
      mask Display: disp('Sensor\n P1')
  Subsystem6 : Subsystem
      mask Display: disp('Pump')
  Subsystem7 : Subsystem
      mask Display: disp('Sensor\n y1')
  Subsystem8 : Subsystem
      mask Display: disp('TANK 2')
  Subsystem9 : Subsystem
      mask Display: disp('OPERATOR\nSET')
  mQp : Outport
  mUb : Outport  Port=2
  "Uo " : Outport  Port=3
  my1 : Outport  Port=4
  my2 : Outport  Port=5
  h1c : Outport  Port=6
  mUp : Outport  Port=7
  mq0 : Outport  Port=8
  y1 : Outport  Port=9
  vol1 : Outport  Port=10
  y2 : Outport  Port=11
  vol2 : Outport  Port=12
  mP1 : Outport  Port=13
  mP2 : Outport  Port=14
  wires:
  Subsystem12/1(mUb) -> mUb/1
  Subsystem3/1(Qv0) -> mq0/1, Subsystem8/1(Qvo)
  Constant/1 -> Subsystem3/3(y0)
  Subsystem13/1(mUp) -> mUp/1
  Subsystem2/1(QVb) -> Subsystem8/2(Qvb), Subsystem1/2(Qvb)
  Subsystem11/1(mUp) -> Subsystem13/1(Up), Subsystem6/1(Up)
  Subsystem9/1(Out3) -> Subsystem11/1(h1c), h1c/1
  Subsystem9/2(Out1) -> "Uo "/1, Subsystem3/1(U0)
  Subsystem7/1(Out5) -> Subsystem11/2(my1), my1/1
  Subsystem14/1(mQp) -> mQp/1
  Subsystem4/1(Out5) -> Subsystem12/1(Ub), Subsystem2/1(Ub)
  Subsystem10/1(my2) -> my2/1, Subsystem4/1(In2)
  Subsystem6/1(mUp) -> Subsystem1/1(Qp), Subsystem14/1(Qp)
  Subsystem7/2(Out1) -> y1/1
  Subsystem7/3(Out2) -> vol1/1
  Subsystem10/2(yy2) -> y2/1
  Subsystem10/3(vol2) -> vol2/1
  Subsystem1/1(y1) -> Subsystem5/1(y1), Subsystem2/2(y1), Subsystem7/1(In1)
  Subsystem5/1(mP1) -> mP1/1
  Subsystem15/1(mP2) -> mP2/1
  Subsystem8/1(y2) -> Subsystem3/2(y2), Subsystem15/1(y2), Subsystem2/3(y2), Subsystem10/1(y2)

== system CHEM_FULL_BENCHMARK/my2 fault/Process ==
  note: y2
  note: y1
  note: Ub
  note: Up
  note: Qvo
      | To users
  note: Qp
  note: Qvb
  Constant : Constant  Value=yo
  Subsystem1 : Subsystem
      mask Display: disp('TANK 1')
  Subsystem10 : Subsystem
      mask Display: disp('Sensor\n y2')
  Subsystem11 : Subsystem
      mask Display: disp('Controller 1')
  Subsystem12 : Subsystem
      mask Display: disp('Sensor\n Ub')
  Subsystem13 : Subsystem
      mask Display: disp('Sensor\n Up')
  Subsystem14 : Subsystem
      mask Display: disp('Sensor\n Qp')
  Subsystem15 : Subsystem
      mask Display: disp('Sensor\n P2')
  Subsystem2 : Subsystem
      mask Display: disp('Valve B')
  Subsystem3 : Subsystem
      mask Display: disp('Valve O')
  Subsystem4 : Subsystem
      mask Display: disp('Controller2')
  Subsystem5 : Subsystem
      mask Display: disp('Sensor\n P1')
  Subsystem6 : Subsystem
      mask Display: disp('Pump')
  Subsystem7 : Subsystem
      mask Display: disp('Sensor\n y1')
  Subsystem8 : Subsystem
      mask Display: disp('TANK 2')
  Subsystem9 : Subsystem
      mask Display: disp('OPERATOR\nSET')
  mQp : Outport
  mUb : Outport  Port=2
  "Uo " : Outport  Port=3
  my1 : Outport  Port=4
  my2 : Outport  Port=5
  h1c : Outport  Port=6
  mUp : Outport  Port=7
  mq0 : Outport  Port=8
  y1 : Outport  Port=9
  vol1 : Outport  Port=10
  y2 : Outport  Port=11
  vol2 : Outport  Port=12
  mP1 : Outport  Port=13
  mP2 : Outport  Port=14
  wires:
  Subsystem12/1(mUb) -> mUb/1
  Subsystem3/1(Qv0) -> mq0/1, Subsystem8/1(Qvo)
  Constant/1 -> Subsystem3/3(y0)
  Subsystem13/1(mUp) -> mUp/1
  Subsystem2/1(QVb) -> Subsystem8/2(Qvb), Subsystem1/2(Qvb)
  Subsystem11/1(mUp) -> Subsystem13/1(Up), Subsystem6/1(Up)
  Subsystem9/1(Out3) -> Subsystem11/1(h1c), h1c/1
  Subsystem9/2(Out1) -> "Uo "/1, Subsystem3/1(U0)
  Subsystem7/1(Out5) -> Subsystem11/2(my1), my1/1
  Subsystem14/1(mQp) -> mQp/1
  Subsystem4/1(Out5) -> Subsystem12/1(Ub), Subsystem2/1(Ub)
  Subsystem10/1(my2) -> my2/1, Subsystem4/1(In2)
  Subsystem6/1(mUp) -> Subsystem1/1(Qp), Subsystem14/1(Qp)
  Subsystem7/2(Out1) -> y1/1
  Subsystem7/3(Out2) -> vol1/1
  Subsystem10/2(yy2) -> y2/1
  Subsystem10/3(vol2) -> vol2/1
  Subsystem5/1(mP1) -> mP1/1
  Subsystem1/1(y1) -> Subsystem5/1(y1), Subsystem2/2(y1), Subsystem7/1(In1)
  Subsystem15/1(mP2) -> mP2/1
  Subsystem8/1(y2) -> Subsystem3/2(y2), Subsystem15/1(y2), Subsystem2/3(y2), Subsystem10/1(y2)

== system CHEM_FULL_BENCHMARK/pump fault/Process ==
  note: y2
  note: y1
  note: Ub
  note: Up
  note: Qvo
      | To users
  note: Qp
  note: Qvb
  Constant : Constant  Value=yo
  Subsystem1 : Subsystem
      mask Display: disp('TANK 1')
  Subsystem10 : Subsystem
      mask Display: disp('Sensor\n y2')
  Subsystem11 : Subsystem
      mask Display: disp('Controller 1')
  Subsystem12 : Subsystem
      mask Display: disp('Sensor\n Ub')
  Subsystem13 : Subsystem
      mask Display: disp('Sensor\n Up')
  Subsystem14 : Subsystem
      mask Display: disp('Sensor\n Qp')
  Subsystem15 : Subsystem
      mask Display: disp('Sensor\n P2')
  Subsystem2 : Subsystem
      mask Display: disp('Valve B')
  Subsystem3 : Subsystem
      mask Display: disp('Valve O')
  Subsystem4 : Subsystem
      mask Display: disp('Controller2')
  Subsystem5 : Subsystem
      mask Display: disp('Sensor\n P1')
  Subsystem6 : Subsystem
      mask Display: disp('Pump')
  Subsystem7 : Subsystem
      mask Display: disp('Sensor\n y1')
  Subsystem8 : Subsystem
      mask Display: disp('TANK 2')
  Subsystem9 : Subsystem
      mask Display: disp('OPERATOR\nSET')
  mQp : Outport
  mUb : Outport  Port=2
  "Uo " : Outport  Port=3
  my1 : Outport  Port=4
  my2 : Outport  Port=5
  h1c : Outport  Port=6
  mUp : Outport  Port=7
  mq0 : Outport  Port=8
  y1 : Outport  Port=9
  vol1 : Outport  Port=10
  y2 : Outport  Port=11
  vol2 : Outport  Port=12
  mP1 : Outport  Port=13
  mP2 : Outport  Port=14
  wires:
  Subsystem12/1(mUb) -> mUb/1
  Subsystem3/1(Qv0) -> mq0/1, Subsystem8/1(Qvo)
  Constant/1 -> Subsystem3/3(y0)
  Subsystem13/1(mUp) -> mUp/1
  Subsystem2/1(QVb) -> Subsystem8/2(Qvb), Subsystem1/2(Qvb)
  Subsystem11/1(mUp) -> Subsystem13/1(Up), Subsystem6/1(Up)
  Subsystem9/1(Out3) -> Subsystem11/1(h1c), h1c/1
  Subsystem9/2(Out1) -> "Uo "/1, Subsystem3/1(U0)
  Subsystem7/1(Out5) -> Subsystem11/2(my1), my1/1
  Subsystem14/1(mQp) -> mQp/1
  Subsystem4/1(Out5) -> Subsystem12/1(Ub), Subsystem2/1(Ub)
  Subsystem10/1(my2) -> my2/1, Subsystem4/1(In2)
  Subsystem6/1(mUp) -> Subsystem1/1(Qp), Subsystem14/1(Qp)
  Subsystem7/2(Out1) -> y1/1
  Subsystem7/3(Out2) -> vol1/1
  Subsystem10/2(yy2) -> y2/1
  Subsystem10/3(vol2) -> vol2/1
  Subsystem1/1(y1) -> Subsystem5/1(y1), Subsystem2/2(y1), Subsystem7/1(In1)
  Subsystem5/1(mP1) -> mP1/1
  Subsystem15/1(mP2) -> mP2/1
  Subsystem8/1(y2) -> Subsystem3/2(y2), Subsystem15/1(y2), Subsystem2/3(y2), Subsystem10/1(y2)

== system CHEM_FULL_BENCHMARK/Empty T2 no leak/Process/Subsystem1 ==
  note: TANK T1 SIMULATION
  note: Qf1
  note: Faultless mode
  note: Faulty mode
      | water leak
  Qp : Inport
  Qvb : Inport  Port=2
  Clock2 : Clock
  Constant : Constant  Value=0
  Constant2 : Constant  Value=0
  Gain : Gain  Gain=1/A1  SaturateOnIntegerOverflow=on  OutDataTypeStr=Inherit: Same as input  ParamDataTypeStr=Inherit: Same as input
  Integrator2 : Integrator  InitialCondition=h1c_0
  Saturation1 : Saturate  UpperLimit=h1max  LowerLimit=0  LinearizeAsGain=off
  Selector : ManualSwitch  CurrentSetting=0
  Sum2 : Sum  Inputs=+--  SaturateOnIntegerOverflow=on  InputSameDT=on  OutDataTypeStr=Inherit: Same as first input
  Switch1 : Switch  Threshold=80  SaturateOnIntegerOverflow=on  InputSameDT=on
  Switch4 : Switch  Threshold=40  SaturateOnIntegerOverflow=on  InputSameDT=on
  flow leak : Constant  Value=Qf1
  y1 : Outport  InitialOutput=0
  wires:
  Gain/1 -> Integrator2/1
  Sum2/1 -> Gain/1
  Qp/1 -> Sum2/1
  Qvb/1 -> Sum2/2
  Clock2/1 -> Switch4/2, Switch1/2
  flow leak/1 -> Switch4/1
  Constant/1 -> Switch4/3, Switch1/1
  Switch4/1 -> Switch1/3
  Selector/1 -> Sum2/3
  Switch1/1 -> Selector/1
  Constant2/1 -> Selector/2
  Integrator2/1 -> Saturation1/1
  Saturation1/1 -> y1/1

== system CHEM_FULL_BENCHMARK/Empty T2 no leak/Process/Subsystem10 ==
  note: SIMULATION OF THE SENSOR y2
  note: Faultless mode
  note: Faulty mode
  note: Faultless mode
  note: Faulty mode
      | water leak
  note: Faultless mode
  note: Faulty mode
      | water leak
  y2 : Inport
  mQo : Inport  Port=2
  Clock1 : Clock
  Clock2 : Clock
  Clock3 : Clock
  Commande vanne 1 : ManualSwitch
  Commande vanne 2 : ManualSwitch
  Commande vanne 3 : ManualSwitch
  Constant{,1,3..4,6} (5 alike) : Constant  Value=0
  Gain : Gain  Gain=1/A2  SaturateOnIntegerOverflow=on  OutDataTypeStr=Inherit: Same as input  ParamDataTypeStr=Inherit: Same as input
  Integrator1 : Integrator
  Integrator2 : Integrator
  Missing Volume : Scope
  Mux : Mux  Inputs=2
  Sum1 : Sum  SaturateOnIntegerOverflow=on  InputSameDT=on  OutDataTypeStr=Inherit: Same as first input
  Sum6 : Sum  SaturateOnIntegerOverflow=on  InputSameDT=on  OutDataTypeStr=Inherit: Same as first input
  Switch1 : Switch  Threshold=40  SaturateOnIntegerOverflow=on  InputSameDT=on
  Switch2 : Switch  Threshold=120  SaturateOnIntegerOverflow=on  InputSameDT=on
  Switch3 : Switch  Threshold=40  SaturateOnIntegerOverflow=on  InputSameDT=on
  Switch4 : Switch  Threshold=120  SaturateOnIntegerOverflow=on  InputSameDT=on
  Switch5 : Switch  Threshold=120  SaturateOnIntegerOverflow=on  InputSameDT=on
  Switch6 : Switch  Threshold=40  SaturateOnIntegerOverflow=on  InputSameDT=on
  my2 noise : UniformRandomNumber  Minimum=-rate_noise_my2  Maximum=rate_noise_my2  Seed=seed  SampleTime=0
  "real and false level " : Scope
  my2 : Outport  InitialOutput=0
  yy2 : Outport  Port=2  InitialOutput=0
  vol2 : Outport  Port=3  InitialOutput=0
  wires:
  my2 noise/1 -> Sum6/2
  Commande vanne 2/1 -> Sum6/1
  y2/1 -> Commande vanne 2/1, Switch1/3, Switch4/1
  Switch4/1 -> Commande vanne 2/2
  Switch1/1 -> Switch4/3
  Constant1/1 -> Switch1/1
  Clock2/1 -> Switch4/2, Switch1/2
  Clock1/1 -> Switch3/2, Switch2/2
  Constant/1 -> Switch3/3, Switch2/1
  Switch3/1 -> Switch2/3
  Switch2/1 -> Commande vanne 1/1
  Constant3/1 -> Commande vanne 1/2
  Sum6/1 -> yy2/1, Mux/2, Sum1/1
  Sum1/1 -> Mux/1, my2/1
  Integrator2/1 -> Gain/1
  Mux/1 -> "real and false level "/1
  Commande vanne 1/1 -> Integrator2/1
  Gain/1 -> Sum1/2
  Clock3/1 -> Switch6/2, Switch5/2
  mQo/1 -> Switch6/1, Switch3/1
  Constant4/1 -> Switch6/3, Switch5/1
  Switch6/1 -> Switch5/3
  Switch5/1 -> Commande vanne 3/1
  Constant6/1 -> Commande vanne 3/2
  Integrator1/1 -> vol2/1, Missing Volume/1
  Commande vanne 3/1 -> Integrator1/1

== system CHEM_FULL_BENCHMARK/Empty T2 no leak/Process/Subsystem11 ==
  note: Faultless mode
  note: Faulty mode
  note: Up
  note: SIMULATION OF THE DIGITAL PI CONTROLLER
  h1c : Inport
  my1 : Inport  Port=2
  Clock2 : Clock
  Commande vanne 2 : ManualSwitch
  Constant1 : Constant  Value=0
  Digital PIController : DiscreteTransferFcn  Numerator=[(Ki*Te+Kp) -Kp]  Denominator=[1 -1]
  Sum : Sum  Inputs=+-  SaturateOnIntegerOverflow=on  InputSameDT=on  OutDataTypeStr=Inherit: Same as first input
  Switch1 : Switch  Threshold=40  SaturateOnIntegerOverflow=on  InputSameDT=on
  Switch4 : Switch  Threshold=120  SaturateOnIntegerOverflow=on  InputSameDT=on
  Zero-Order Hold4 : ZeroOrderHold  SampleTime=-1
  mUp : Outport  InitialOutput=0
  wires:
  Switch4/1 -> Commande vanne 2/2
  Commande vanne 2/1 -> mUp/1
  Digital PIController/1 -> Switch1/3, Switch4/1, Commande vanne 2/1
  Switch1/1 -> Switch4/3
  Constant1/1 -> Switch1/1
  Clock2/1 -> Switch4/2, Switch1/2
  h1c/1 -> Sum/1
  my1/1 -> Sum/2
  Zero-Order Hold4/1 -> Digital PIController/1
  Sum/1 -> Zero-Order Hold4/1

== system CHEM_FULL_BENCHMARK/Empty T2 no leak/Process/Subsystem12 ==
  note: SIMULATION OF THE SENSOR Ub
  note: Faultless mode
  note: Faulty mode
  Ub : Inport
  Clock2 : Clock
  Commande vanne 2 : ManualSwitch
  Constant1 : Constant  Value=0
  Switch1 : Switch  Threshold=40  SaturateOnIntegerOverflow=on  InputSameDT=on
  Switch4 : Switch  Threshold=120  SaturateOnIntegerOverflow=on  InputSameDT=on
  mUb : Outport  InitialOutput=0
  wires:
  Clock2/1 -> Switch1/2, Switch4/2
  Constant1/1 -> Switch1/1
  Switch1/1 -> Switch4/3
  Switch4/1 -> Commande vanne 2/2
  Ub/1 -> Commande vanne 2/1, Switch1/3, Switch4/1
  Commande vanne 2/1 -> mUb/1
